simulink model "SMCsim"  (R2024b)
settings: Solver=VariableStepAuto  StartTime=0.0  StopTime=10.0  RelTol=1e-3
values from neighbouring files (symbols this model uses):
  Kr_SMC = 0.5    [SMCpuresetup.m]    (also in smcpure1.m)
  Ksw_SMC = 1.5    [SMC_Setup.m]    (also in SMC_Tracking_Setup.m = 1; SMCpuresetup.m = 1; smcpure1.m = 1)
  phi_SMC = 0.05    [SMC_Setup.m]    (also in SMC_Tracking_Setup.m; SMCpuresetup.m; smcpure1.m)
  S_SMC = K_Nom_LQR_Br    [SMC_Setup.m]    (also in SMC_Tracking_Setup.m; SMCpuresetup.m = [1.0, 25.0, 0.8, 3.0]; smcpure1.m = [0, lambda_theta_SMC, 0, 1])
  uMax_SMC = drv.Vbus    [SMC_Setup.m]    (also in SMC_Tracking_Setup.m; SMCpuresetup.m; smcpure1.m)
undefined symbols (not defined in the file or in its folder): A, B, C_filter, drv, dspblkCoreblockFVToolHelper, gbox, gcbh, sens, T, Ts
settings Model: Creator=marja  LastModifiedBy=marja

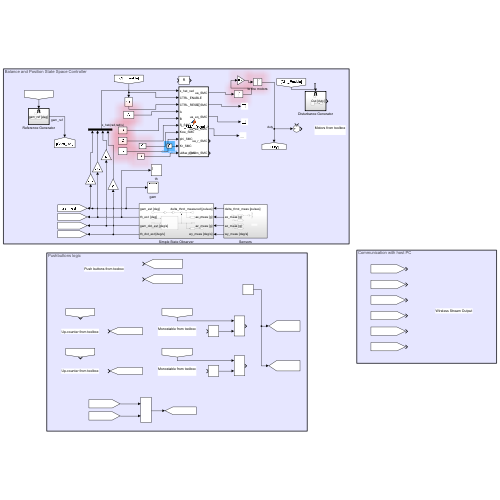
[thumbnail: Simulink's stored preview of the top-level diagram]
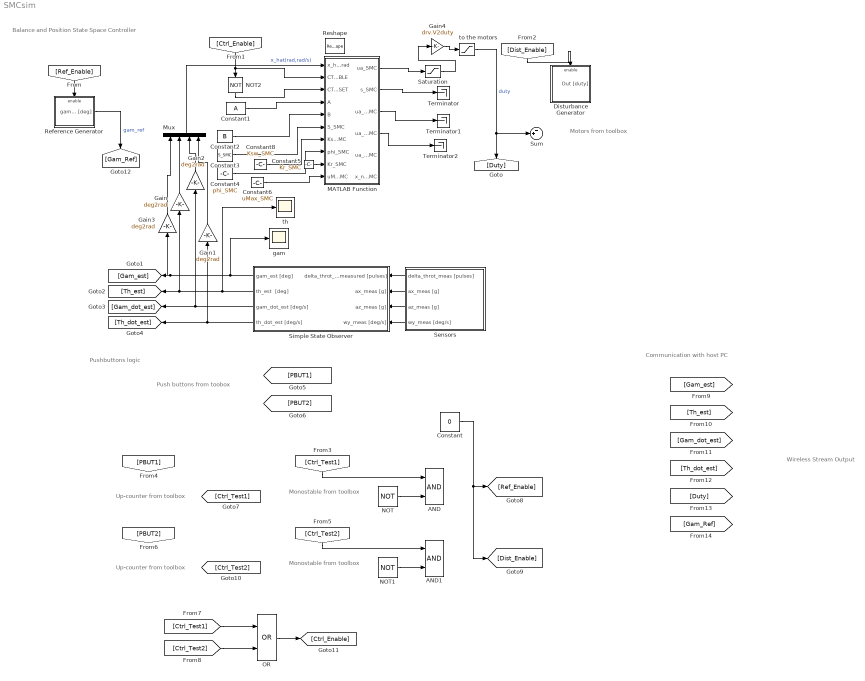
== system SMCsim ==
  note: Monostable from toolbox
  note: Push buttons from toobox
  note: Up-counter from toolbox
  note: Monostable from toolbox
  note: Communication with host PC
  note: Motors from toolbox
  note: Wireless Stream Output
  note: Balance and Position State Space Controller
  note: Up-counter from toolbox
  note: Pushbuttons logic
  AND : Logic  AllPortsSameDT=off  OutDataTypeStr=boolean
  AND1 : Logic  AllPortsSameDT=off  OutDataTypeStr=boolean
  Constant : Constant  Value=0  SampleTime=0.01
  Constant1 : Constant  Value=A  SampleTime=Ts
  Constant2 : Constant  Value=B  SampleTime=Ts
  Constant3 : Constant  Value=S_SMC  SampleTime=Ts
  Constant4 : Constant  Value=phi_SMC  SampleTime=Ts
  Constant5 : Constant  Value=Kr_SMC  SampleTime=Ts
  Constant6 : Constant  Value=uMax_SMC  SampleTime=Ts
  Constant8 : Constant  Value=Ksw_SMC  SampleTime=Ts
  Disturbance Generator : Subsystem
  Gain{,1..3} (4 alike) : Gain  Gain=deg2rad
  Gain4 : Gain  Gain=drv.V2duty
  MATLAB Function : MATLAB Function  TreatAsAtomicUnit=on
  Mux : Mux
  NOT : Logic  Operator=NOT  AllPortsSameDT=off  OutDataTypeStr=boolean
  NOT1 : Logic  Operator=NOT  AllPortsSameDT=off  OutDataTypeStr=boolean
  NOT2 : Logic  Operator=NOT  AllPortsSameDT=off  OutDataTypeStr=boolean
  OR : Logic  Operator=OR  AllPortsSameDT=off  OutDataTypeStr=boolean
  Reference Generator : Subsystem
  Reshape : Reshape  OutputDimensionality=Customize  OutputDimensions=[4,1]
  Saturation : Saturate  UpperLimit=+drv.Vbus  LowerLimit=-drv.Vbus
  Sensors : Subsystem
  Simple State Observer : Subsystem
  Sum : Sum  Inputs=-+|
  Terminator : Terminator
  Terminator1 : Terminator
  Terminator2 : Terminator
  gam : Scope
  th : Scope
  to the motors : Saturate  UpperLimit=drv.dutymax  LowerLimit=-drv.dutymax
  wires:
  Gain/1 -> Mux/2
  OR/1 -> [Ctrl_Enable]
  Gain2/1 -> Mux/3
  Reference Generator/1(gam_ref [deg]) -> [Gam_Ref]  "gam_ref"
  Constant/1 -> [Dist_Enable], [Ref_Enable]
  Simple State Observer/4(th_dot_est [deg/s]) -> [Th_dot_est], Gain1/1
  [Dist_Enable] -> Disturbance Generator/Enable
  [Ctrl_Test2] -> OR/2
  Saturation/1 -> Gain4/1
  Simple State Observer/2(th_est  [deg]) -> th/1, Gain/1, [Th_est]
  Gain1/1 -> Mux/4
  Sensors/1(delta_throt_meas [pulses]) -> Simple State Observer/1(delta_throt_measured [pulses])
  [Ctrl_Test2] -> AND1/1
  NOT1/1 -> AND1/2
  Simple State Observer/3(gam_dot_est [deg/s]) -> [Gam_dot_est], Gain2/1
  Simple State Observer/1(gam_est [deg]) -> gam/1, Gain3/1, [Gam_est]
  Gain4/1 -> to the motors/1
  Sensors/4(wy_meas [deg/s]) -> Simple State Observer/4(wy_meas [deg/s])
  to the motors/1 -> Sum/2, [Duty]  "duty"
  Gain3/1 -> Mux/1
  [Ctrl_Test1] -> AND/1
  [Ctrl_Test1] -> OR/1
  [Ctrl_Enable] -> MATLAB Function/2(CTRL_ENABLE), NOT2/1
  [Ref_Enable] -> Reference Generator/Enable
  Sensors/3(az_meas [g]) -> Simple State Observer/3(az_meas [g])
  Sensors/2(ax_meas [g]) -> Simple State Observer/2(ax_meas [g])
  NOT/1 -> AND/2
  Mux/1 -> MATLAB Function/1(x_hat_rad)  "x_hat(rad,rad/s)"
  NOT2/1 -> MATLAB Function/3(CTRL_RESET)
  Constant1/1 -> MATLAB Function/4(A)
  Constant2/1 -> MATLAB Function/5(B)
  Constant3/1 -> MATLAB Function/6(S_SMC)
  Constant8/1 -> MATLAB Function/7(Ksw_SMC)
  Constant4/1 -> MATLAB Function/8(phi_SMC)
  Constant6/1 -> MATLAB Function/10(uMax_SMC)
  MATLAB Function/1(ua_SMC) -> Saturation/1
  MATLAB Function/2(s_SMC) -> Terminator/1
  MATLAB Function/3(ua_eq_SMC) -> Terminator1/1
  MATLAB Function/4(ua_sw_SMC) -> Terminator2/1
  Constant5/1 -> MATLAB Function/9(Kr_SMC)

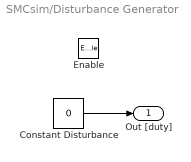
== system SMCsim/Disturbance Generator ==
  Enable : EnablePort
  Constant Disturbance : Constant  Value=0
  Out [duty] : Outport  OutputWhenDisabled=reset  InitialOutput=0
  wires:
  Constant Disturbance/1 -> Out [duty]/1

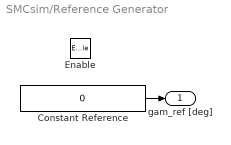
== system SMCsim/Reference Generator ==
  Enable : EnablePort
  Constant Reference : Constant  Value=0
  gam_ref [deg] : Outport  OutputWhenDisabled=reset  InitialOutput=0
  wires:
  Constant Reference/1 -> gam_ref [deg]/1

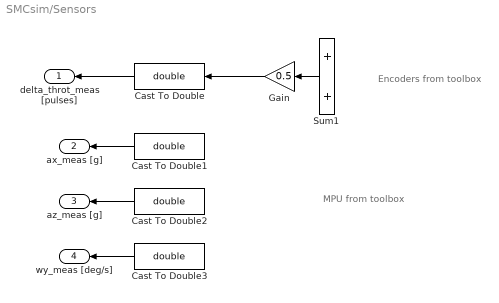
== system SMCsim/Sensors ==
  note: Encoders from toolbox
  note: MPU from toolbox
  Cast To Double{,1..3} (4 alike) : DataTypeConversion  OutDataTypeStr=double  SaturateOnIntegerOverflow=off  RndMeth=Floor
  Gain : Gain  Gain=0.5
  Sum1 : Sum
  delta_throt_meas [pulses] : Outport
  ax_meas [g] : Outport  Port=2
  az_meas [g] : Outport  Port=3
  wy_meas [deg/s] : Outport  Port=4
  wires:
  Sum1/1 -> Gain/1
  Gain/1 -> Cast To Double/1
  Cast To Double/1 -> delta_throt_meas [pulses]/1
  Cast To Double3/1 -> wy_meas [deg/s]/1
  Cast To Double2/1 -> az_meas [g]/1
  Cast To Double1/1 -> ax_meas [g]/1

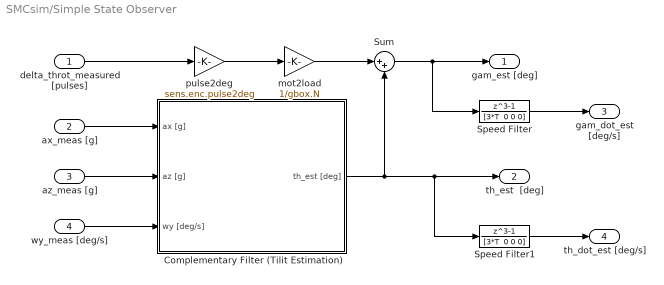
== system SMCsim/Simple State Observer ==
  delta_throt_measured [pulses] : Inport
  ax_meas [g] : Inport  Port=2
  az_meas [g] : Inport  Port=3
  wy_meas [deg/s] : Inport  Port=4
  Complementary Filter (Tilit Estimation) : Subsystem
  Speed Filter : DiscreteTransferFcn  LoadFcn=dspblkCoreblockFVToolHelper(gcbh,'load');  Numerator=[1 0 0 -1]  Denominator="[3*T  0 0 0]"
      settings: CopyFcn=dspblkCoreblockFVToolHelper(gcbh,'copy');  DeleteFcn=dspblkCoreblockFVToolHelper(gcbh,'close');  ModelCloseFcn=dspblkCoreblockFVToolHelper(gcbh,'close');  PreSaveFcn=dspblkCoreblockFVToolHelper(gcbh,'presave');  PostSaveFcn=dspblkCoreblockFVToolHelper(gcbh,'postsave');  CloseFcn=dspblkCoreblockFVToolHelper(gcbh,'close');
  Speed Filter1 : DiscreteTransferFcn  LoadFcn=dspblkCoreblockFVToolHelper(gcbh,'load');  Numerator=[1 0 0 -1]  Denominator="[3*T  0 0 0]"
      settings: CopyFcn=dspblkCoreblockFVToolHelper(gcbh,'copy');  DeleteFcn=dspblkCoreblockFVToolHelper(gcbh,'close');  ModelCloseFcn=dspblkCoreblockFVToolHelper(gcbh,'close');  PreSaveFcn=dspblkCoreblockFVToolHelper(gcbh,'presave');  PostSaveFcn=dspblkCoreblockFVToolHelper(gcbh,'postsave');  CloseFcn=dspblkCoreblockFVToolHelper(gcbh,'close');
  Sum : Sum  Inputs=|++
  mot2load : Gain  Gain=1/gbox.N
  pulse2deg : Gain  Gain=sens.enc.pulse2deg
  gam_est [deg] : Outport
  th_est  [deg] : Outport  Port=2
  gam_dot_est [deg/s] : Outport  Port=3
  th_dot_est [deg/s] : Outport  Port=4
  wires:
  mot2load/1 -> Sum/1
  Complementary Filter (Tilit Estimation)/1(th_est [deg]) -> th_est  [deg]/1, Speed Filter1/1, Sum/2
  Speed Filter1/1 -> th_dot_est [deg/s]/1
  delta_throt_measured [pulses]/1 -> pulse2deg/1
  Speed Filter/1 -> gam_dot_est [deg/s]/1
  pulse2deg/1 -> mot2load/1
  Sum/1 -> gam_est [deg]/1, Speed Filter/1
  ax_meas [g]/1 -> Complementary Filter (Tilit Estimation)/1(ax [g])
  az_meas [g]/1 -> Complementary Filter (Tilit Estimation)/2(az [g])
  wy_meas [deg/s]/1 -> Complementary Filter (Tilit Estimation)/3(wy [deg/s])

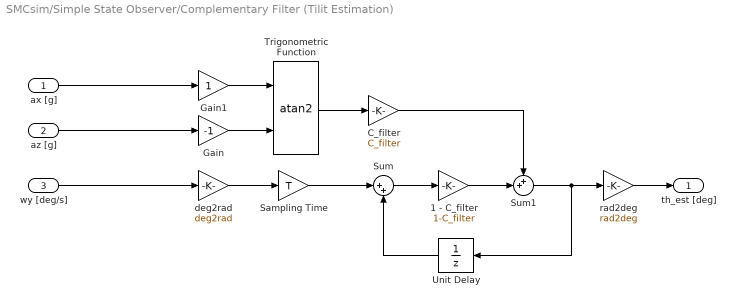
== system SMCsim/Simple State Observer/Complementary Filter (Tilit Estimation) ==
  ax [g] : Inport
  az [g] : Inport  Port=2
  wy [deg/s] : Inport  Port=3
  1 - C_filter : Gain  Gain=1-C_filter
  C_filter : Gain  Gain=C_filter
  Gain : Gain  Gain=-1
  Gain1 : Gain
  Sampling Time : Gain  Gain=T
  Sum : Sum  Inputs=|++
  Sum1 : Sum  Inputs=++|
  Trigonometric Function : Trigonometry  Operator=atan2
  Unit Delay : UnitDelay  SampleTime=T  HasFrameUpgradeWarning=on
  deg2rad : Gain  Gain=deg2rad
  rad2deg : Gain  Gain=rad2deg
  th_est [deg] : Outport
  wires:
  Trigonometric Function/1 -> C_filter/1
  Gain/1 -> Trigonometric Function/2
  rad2deg/1 -> th_est [deg]/1
  deg2rad/1 -> Sampling Time/1
  Sum/1 -> 1 - C_filter/1
  Gain1/1 -> Trigonometric Function/1
  Sum1/1 -> Unit Delay/1, rad2deg/1
  Sampling Time/1 -> Sum/1
  1 - C_filter/1 -> Sum1/2
  Unit Delay/1 -> Sum/2
  C_filter/1 -> Sum1/1
  ax [g]/1 -> Gain1/1
  az [g]/1 -> Gain/1
  wy [deg/s]/1 -> deg2rad/1

== matlab function SMCsim/MATLAB Function ==
  data: x_hat_rad input; ua_SMC output; CTRL_ENABLE input; CTRL_RESET input; A input; B input; S_SMC input; Ksw_SMC input; phi_SMC input; Kr_SMC input; uMax_SMC input; s_SMC output; ua_eq_SMC output; ua_sw_SMC output; ua_r_SMC output; x_norm_SMC output
function [ua_SMC,s_SMC,ua_eq_SMC,ua_sw_SMC,ua_r_SMC,x_norm_SMC] = Pure_SMC_Regulator( ...
    x_hat_rad, CTRL_ENABLE, CTRL_RESET, ...
    A, B, S_SMC, Ksw_SMC, phi_SMC, Kr_SMC, uMax_SMC)
%#codegen
% Pure periodic Sliding Mode Controller for balancing robot.
% NO reference tracking.
%
% State:
%   x_hat_rad = [gamma; theta; gamma_dot; theta_dot]
% units:
%   [rad; rad; rad/s; rad/s]
%
% Linear model:
%   x_dot = A*x + B*ua
%
% Sliding variable:
%   s = S_SMC*x
%
% Pure SMC law:
%   ua = ua_eq + ua_r + ua_sw
%
% where:
%   ua_eq = -(S*A*x)/(S*B)
%   ua_r  = -Kr*s/(S*B)
%   ua_sw = -Ksw*sat(s/phi)

%% Safe output when disabled or reset
if CTRL_RESET || ~CTRL_ENABLE
    ua_SMC = 0;
    s_SMC = 0;
    ua_eq_SMC = 0;
    ua_sw_SMC = 0;
    ua_r_SMC = 0;
    x_norm_SMC = 0;
    return;
end

%% State norm for logging/debugging
x_norm_SMC = sqrt(x_hat_rad.'*x_hat_rad);

%% Sliding variable
s_SMC = S_SMC*x_hat_rad;

%% S*B
SB_SMC = S_SMC*B;

if abs(SB_SMC) < 1e-6
    ua_eq_SMC = 0;
    ua_r_SMC = 0;
else
    %% Equivalent control
    % Makes s_dot = 0 in the nominal linear model, ignoring switching.
    ua_eq_SMC = -(S_SMC*A*x_hat_rad)/SB_SMC;

    %% Reaching-rate term
    % Adds smooth convergence of s toward zero.
    ua_r_SMC = -(Kr_SMC*s_SMC)/SB_SMC;
end

%% Saturation approximation of sign(s)
if phi_SMC < 1e-6
    phi_use_SMC = 1e-6;
else
    phi_use_SMC = phi_SMC;
end

sat_arg_SMC = s_SMC/phi_use_SMC;

if sat_arg_SMC > 1
    sat_s_SMC = 1;
elseif sat_arg_SMC < -1
    sat_s_SMC = -1;
else
    sat_s_SMC = sat_arg_SMC;
end

%% Switching robust term
ua_sw_SMC = -Ksw_SMC*sat_s_SMC;

%% Total motor voltage command
ua_SMC = ua_eq_SMC + ua_r_SMC + ua_sw_SMC;

%% Voltage saturation
if ua_SMC > uMax_SMC
    ua_SMC = uMax_SMC;
elseif ua_SMC < -uMax_SMC
    ua_SMC = -uMax_SMC;
end
